simulink subsystem "MqMatrix"  (R2024b)
settings: Solver=VariableStepAuto  StartTime=0.0  StopTime=10.0  RelTol=1e-3
values from neighbouring files (symbols this model uses):
  M11 = 2*wheel.Iyy + 2*gbox.N^2*mot.rot.Iyy + (body.m + 2*wheel.m + 2*mot.rot.m)*wheel.r^2    [A_final_results.m]    (also in Plant_balrob_calculations.m = 2*wheel.Iyy + 2 * gbox.N^2*mot.rot.Iyy +      (body.m + 2*wh)
  M22 = body.Iyy + 2*(1-gbox.N)^2 *mot.rot.Iyy + body.m*body.zb^2 + 2*mot.rot.m*mot.rot.zb^2    [A_final_results.m]    (also in Plant_balrob_calculations.m = body.Iyy + 2*(1-gbox.N)^2 *mot.rot.Iyy +      body.m*body.zb)
undefined symbols (not defined in the file or in its folder): body, gbox, mot, wheel
settings Model: Creator=federico  LastModifiedBy=federico

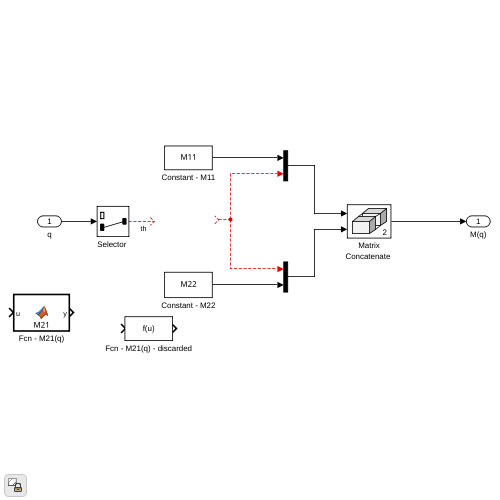
[thumbnail: Simulink's stored preview of the top-level diagram]
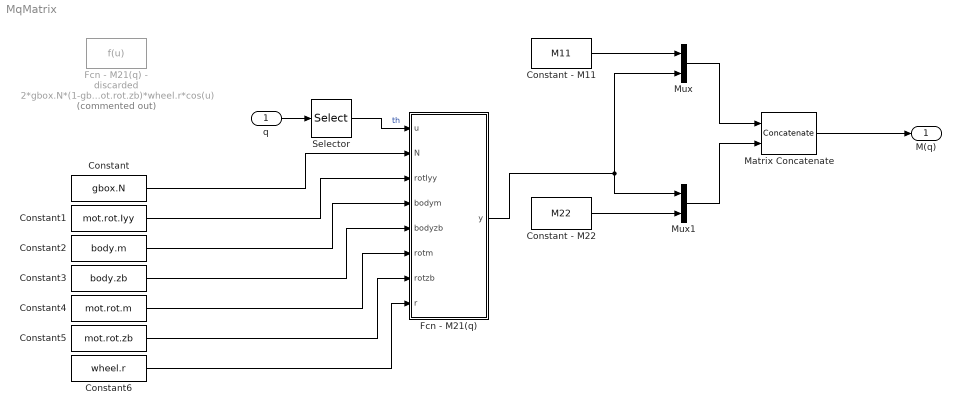
== system MqMatrix ==
  q : Inport
  Constant : Constant  Value=gbox.N
  Constant - M11 : Constant  Value=M11
  Constant - M22 : Constant  Value=M22
  Constant1 : Constant  Value=mot.rot.Iyy
  Constant2 : Constant  Value=body.m
  Constant3 : Constant  Value=body.zb
  Constant4 : Constant  Value=mot.rot.m
  Constant5 : Constant  Value=mot.rot.zb
  Constant6 : Constant  Value=wheel.r
  Fcn - M21(q) : MATLAB Function  TreatAsAtomicUnit=on
  Fcn - M21(q) - discarded : Fcn  Commented=on  Expr=2*gbox.N*(1-gbox.N)*mot.rot.Iyy + (body.m*body.zb + 2*mot.rot.m*mot.rot.zb)*wheel.r*cos(u)
  "Matrix Concatenate " : Concatenate  Mode=Multidimensional array  ConcatenateDimension=2
  Mux : Mux  Inputs=2
  Mux1 : Mux  Inputs=2
  "Selector " : Selector  InputPortWidth=2  IndexOptions=Index vector (dialog)  Indices=[2]  OutputSizes=1
  M(q) : Outport
  wires:
  q/1 -> "Selector "/1
  "Selector "/1 -> Fcn - M21(q)/1(u)  "th"
  Constant - M11/1 -> Mux/1
  Fcn - M21(q)/1(y) -> Mux1/1, Mux/2
  Constant - M22/1 -> Mux1/2
  Mux/1 -> "Matrix Concatenate "/1
  Mux1/1 -> "Matrix Concatenate "/2
  "Matrix Concatenate "/1 -> M(q)/1
  Constant6/1 -> Fcn - M21(q)/8(r)
  Constant5/1 -> Fcn - M21(q)/7(rotzb)
  Constant4/1 -> Fcn - M21(q)/6(rotm)
  Constant3/1 -> Fcn - M21(q)/5(bodyzb)
  Constant2/1 -> Fcn - M21(q)/4(bodym)
  Constant1/1 -> Fcn - M21(q)/3(rotIyy)
  Constant/1 -> Fcn - M21(q)/2(N)

== matlab function MqMatrix/Fcn - M21(q) ==
  data: u input; y output; N input; rotIyy input; bodym input; bodyzb input; rotm input; rotzb input; r input
function y = M21(u, N, rotIyy, bodym, bodyzb, rotm, rotzb, r)

y = 2*N*(1-N)*rotIyy + (bodym*bodyzb + 2*rotm*rotzb)*r*cos(u);
